simulink model "position"  (R2016b)
settings: Solver=VariableStepAuto  StartTime=0.0  StopTime=20  RelTol=1e-3
settings Model: Creator=nguyenquoctruong  LastModifiedBy=nguyenquoctruong

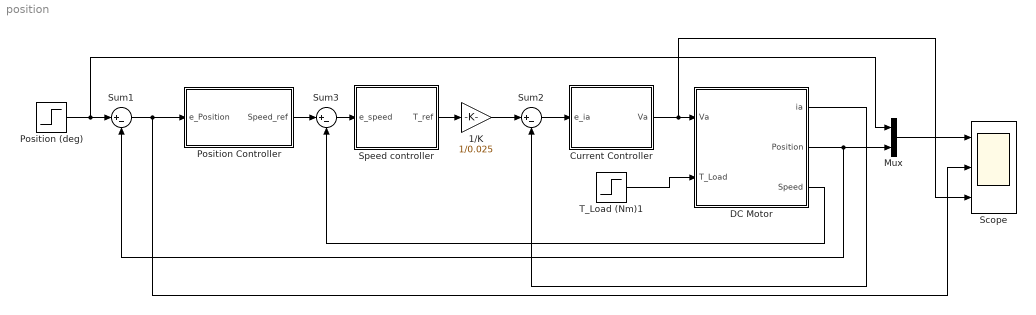
== system position ==
  1/K : Gain  Gain=1/0.025
  Current Controller : Subsystem  mask{Kp=5, Ki=0.004, Vmax=12}
      mask prompts: Vmax "Vmax(V)"
  DC Motor : Subsystem  mask{Ra=0.1, K=0.025, Jm=0.002, La=2*(10^-3), Bm=0.0002}
      mask prompts: Ra "Ra(Ohm)"; K "K(Vs)"; Jm "Jm(kgm^2)"; La "La(H)"; Bm "Bm(Nm.s.rad^-1)"
  Mux : Mux  Inputs=2
  Position (deg) : Step  Time=2.2  After=90  SampleTime=0
  Position Controller : Subsystem  mask{Kp=3, Ki=0, Speedmax=4430}
      mask prompts: Speedmax "Speedmax(rpm)"
  Scope : Scope  NumInputPorts=3
  Speed controller : Subsystem  mask{Kp=10, Ki=0, Tmax=2.66}
      mask prompts: Tmax "Tmax(Nm)"
  Sum1 : Sum  Inputs=|+-
  Sum2 : Sum  Inputs=|+-
  Sum3 : Sum  Inputs=|+-
  T_Load (Nm)1 : Step  Time=12  After=0.5  SampleTime=0
  wires:
  DC Motor/1(ia) -> Sum2/2
  1/K/1 -> Sum2/1
  Sum1/1 -> Scope/2, Position Controller/1(e_Position)
  DC Motor/3("Speed ") -> Sum3/2
  Position Controller/1("Speed_ref ") -> Sum3/1
  Speed controller/1("T_ref ") -> 1/K/1
  Sum3/1 -> Speed controller/1(e_speed)
  Sum2/1 -> Current Controller/1(e_ia)
  Current Controller/1("Va ") -> DC Motor/1("Va "), Scope/3
  Mux/1 -> Scope/1
  Position (deg)/1 -> Mux/1, Sum1/1
  DC Motor/2(Position) -> Mux/2, Sum1/2
  T_Load (Nm)1/1 -> DC Motor/2(T_Load)

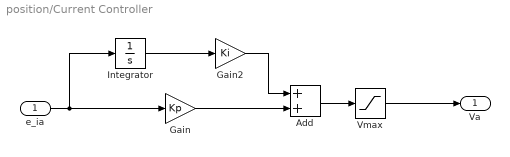
== system position/Current Controller ==
  e_ia : Inport
  Add : Sum
  Gain : Gain  Gain=Kp
  Gain2 : Gain  Gain=Ki
  Integrator : Integrator
  Vmax : Saturate  UpperLimit=Vmax  LowerLimit=-Vmax
  "Va " : Outport
  wires:
  Integrator/1 -> Gain2/1
  e_ia/1 -> Integrator/1, Gain/1
  Gain2/1 -> Add/1
  Add/1 -> Vmax/1
  Vmax/1 -> "Va "/1
  Gain/1 -> Add/2

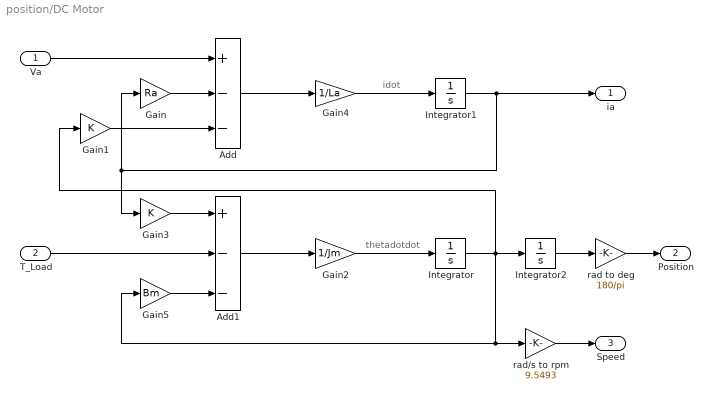
== system position/DC Motor ==
  note: idot
  note: thetadotdot
  "Va " : Inport
  T_Load : Inport  Port=2
  Add : Sum  Inputs=+--
  Add1 : Sum  Inputs=+--
  Gain : Gain  Gain=Ra
  Gain1 : Gain  Gain=K
  Gain2 : Gain  Gain=1/Jm
  Gain3 : Gain  Gain=K
  Gain4 : Gain  Gain=1/La
  Gain5 : Gain  Gain=Bm
  Integrator : Integrator
  Integrator1 : Integrator
  Integrator2 : Integrator
  rad to deg : Gain  Gain=180/pi
  rad/s to rpm : Gain  Gain=9.5493
  ia : Outport
  Position : Outport  Port=2
  "Speed " : Outport  Port=3
  wires:
  rad to deg/1 -> Position/1
  Integrator2/1 -> rad to deg/1
  rad/s to rpm/1 -> "Speed "/1
  Gain5/1 -> Add1/3
  Integrator/1 -> rad/s to rpm/1, Gain5/1, Integrator2/1, Gain1/1
  Integrator1/1 -> Gain3/1, Gain/1, ia/1
  Gain2/1 -> Integrator/1
  Add1/1 -> Gain2/1
  Add/1 -> Gain4/1
  Gain4/1 -> Integrator1/1
  "Va "/1 -> Add/1
  Gain3/1 -> Add1/1
  Gain1/1 -> Add/3
  T_Load/1 -> Add1/2
  Gain/1 -> Add/2

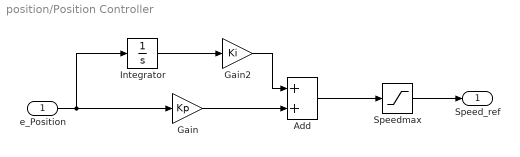
== system position/Position Controller ==
  e_Position : Inport
  Add : Sum
  Gain : Gain  Gain=Kp
  Gain2 : Gain  Gain=Ki
  Integrator : Integrator
  Speedmax : Saturate  UpperLimit=Speedmax  LowerLimit=-Speedmax
  "Speed_ref " : Outport
  wires:
  Add/1 -> Speedmax/1
  Gain2/1 -> Add/1
  Gain/1 -> Add/2
  Integrator/1 -> Gain2/1
  Speedmax/1 -> "Speed_ref "/1
  e_Position/1 -> Gain/1, Integrator/1

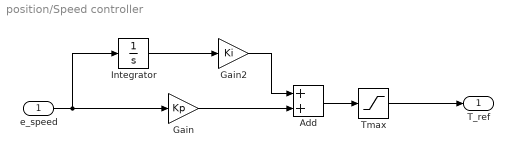
== system position/Speed controller ==
  e_speed : Inport
  Add : Sum
  Gain : Gain  Gain=Kp
  Gain2 : Gain  Gain=Ki
  Integrator : Integrator
  Tmax : Saturate  UpperLimit=Tmax  LowerLimit=-Tmax
  "T_ref " : Outport
  wires:
  Gain/1 -> Add/2
  Tmax/1 -> "T_ref "/1
  Add/1 -> Tmax/1
  Gain2/1 -> Add/1
  e_speed/1 -> Gain/1, Integrator/1
  Integrator/1 -> Gain2/1
